simulink model "P2simulink"  (R2022b)
settings: Solver=VariableStepAuto  StartTime=0.0  StopTime=10.0  RelTol=1e-3
values from neighbouring files (symbols this model uses):
  Altura = 100    [P2.m]    (also in P3.m = 10; P4.m = 10; TestGraph.m = 10; ZenoPlot.m = 10)
  coefAtrito = -0.8    [P2.m]
  K = 0:0.1:1    [P1.m]    (also in P2.m = -1; P4.m = -0.8; TestGraph.m = -0.8; ZenoPlot.m = -0.8)
  V = 0    [P1.m]    (also in P2.m = 15; P3.m = 15; P4.m = 15; QuiverTest.m = zeros(length(U),length(U)) -g)
libraries: simulink x1
settings Model: Creator=TERESA NOGUEIRA  LastModifiedBy=TERESA NOGUEIRA
settings SolverCC: ZeroCrossAlgorithm=Adaptive

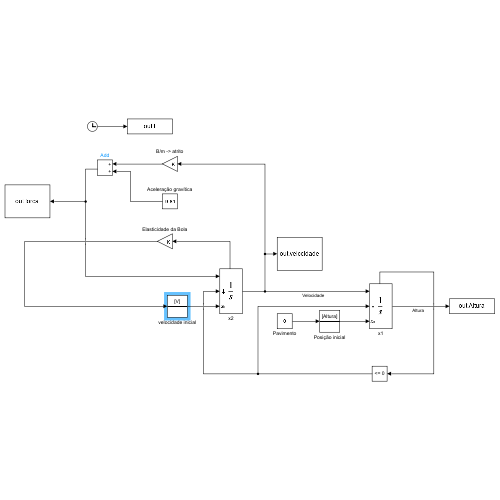
[thumbnail: Simulink's stored preview of the top-level diagram]
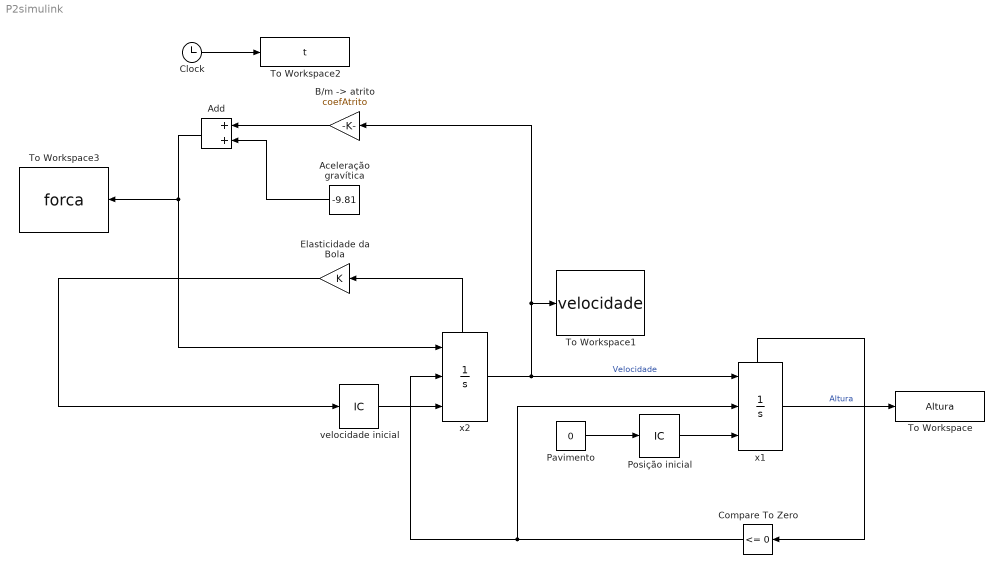
== system P2simulink ==
  Aceleração gravítica : Constant  Value=-9.81
  Add : Sum
  "B/m -> atrito" : Gain  Gain=coefAtrito
  Clock : Clock
      settings: Decimation=200
  Compare To Zero : simulink/Logic and Bit Operations/Compare To Zero  relop=<=  OutDataTypeStr=boolean
  Elasticidade da Bola : Gain  Gain=K
  Pavimento : Constant  Value=0
  Posição inicial : InitialCondition  Value=Altura
  To Workspace : ToWorkspace  VariableName=Altura  SampleTime=-1
      settings: Save2DSignal=2-D array (concatenate along first dimension)
  To Workspace1 : ToWorkspace  VariableName=velocidade  SampleTime=-1
      settings: Save2DSignal=2-D array (concatenate along first dimension)
  To Workspace2 : ToWorkspace  VariableName=t  SampleTime=-1
      settings: Save2DSignal=2-D array (concatenate along first dimension)
  To Workspace3 : ToWorkspace  VariableName=forca  SampleTime=-1
      settings: Save2DSignal=2-D array (concatenate along first dimension)
  velocidade inicial : InitialCondition  Value=V
  x1 : Integrator  ExternalReset=rising  InitialConditionSource=external  ShowStatePort=on
  x2 : Integrator  ExternalReset=rising  InitialConditionSource=external  ShowStatePort=on
  wires:
  x2/1 -> x1/1, "B/m -> atrito"/1, To Workspace1/1  "Velocidade"
  velocidade inicial/1 -> x2/3
  Elasticidade da Bola/1 -> velocidade inicial/1
  Posição inicial/1 -> x1/3
  Clock/1 -> To Workspace2/1
  Pavimento/1 -> Posição inicial/1
  x1/1 -> To Workspace/1  "Altura"
  x2/State -> Elasticidade da Bola/1
  Compare To Zero/1 -> x2/2, x1/2
  x1/State -> Compare To Zero/1
  "B/m -> atrito"/1 -> Add/1
  Aceleração gravítica/1 -> Add/2
  Add/1 -> To Workspace3/1, x2/1
